simulink model "free_msd"  (Simulink 7.8)
settings: Solver=ode4  StartTime=0.0  StopTime=time_span  RelTol=1e-3
undefined symbols (not defined in the file or in its folder): m, outstr, samp_time
settings Model: Creator=Kourosh Danai  LastModifiedBy=BionicBill
settings DebuggingCC: AlgebraicLoopMsg=none  SolverPrmCheckMsg=none  FcnCallInpInsideContextMsg=Use local settings  StrictBusMsg=Warning
settings SFSimCC: SimParseCustomCode=off

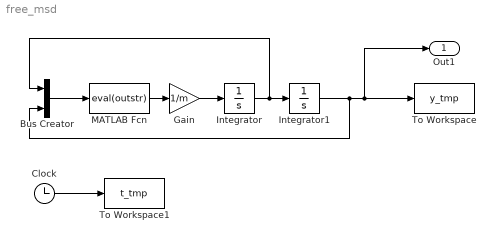
== system free_msd ==
  Bus Creator : BusCreator  Inputs=2
  Clock : Clock
  Gain : Gain  Gain=1/m
  Integrator : Integrator  InitialCondition=0.2
  Integrator1 : Integrator  InitialCondition=0.2
  MATLAB Fcn : MATLABFcn  MATLABFcn=eval(outstr)  SampleTime=samp_time
  To Workspace : ToWorkspace  VariableName=y_tmp  SampleTime=-1  SaveFormat=Array
  To Workspace1 : ToWorkspace  VariableName=t_tmp  SampleTime=-1  SaveFormat=Array
  Out1 : Outport
  wires:
  Integrator/1 -> Integrator1/1, Bus Creator/1
  Bus Creator/1 -> MATLAB Fcn/1
  MATLAB Fcn/1 -> Gain/1
  Gain/1 -> Integrator/1
  Clock/1 -> To Workspace1/1
  Integrator1/1 -> To Workspace/1, Out1/1, Bus Creator/2
